simulink model "CAMFC2_04_Quad_03"  (R2018b)
settings: Solver=ode45  StartTime=0.0  StopTime=600  RelTol=1e-3  EnableMultiTasking=on
InitFcn:
  | constant_CAMFC2_04_Quad_03
values from neighbouring files (symbols this model uses):
  alpha = 0.1    [constant_CAMFC2_01_WMR01.m]    (also in constant_CAMFC2_04_Comp.m = 0.01; constant_CAMFC2_04_Quad_03.m; constant_CAMFC2_04_Simple.m = 0.01; constant_CAMFC2_04_Simple_DoubleIntegrator.m = 0.01)
  AN = [     0 1 0 0 ... (first row only)    [constant_CAMFC2_01_WMR01.m]    (also in constant_CAMFC2_04_Comp.m = [     0 1 0 0 1; constant_CAMFC2_04_Quad_03.m; constant_CAMFC2_04_Simple.m; constant_CAMFC2_04_Simple_DoubleIntegrator.m)
  B = eye(n)    [constant_CAMFC2_01_WMR01.m]    (also in constant_CAMFC2_04_Quad_03.m; constant_CAMFC2_Quad_New_02.m)
  BBT_inv = ((B'*B)^(-1))*B'    [constant_CAMFC2_04_Quad_03.m]    (also in constant_CAMFC2_Quad_New_02.m)
  Beta = 0.2    [constant_CAMFC2_04_Quad_03.m]    (also in constant_CAMFC2_Quad_New_02.m = 0.1)
  BN = [     1 0 0 0 ... (first row only)    [constant_CAMFC2_01_WMR01.m]    (also in constant_CAMFC2_04_Comp.m = [     0 0 0 0 0; constant_CAMFC2_04_Quad_03.m; constant_CAMFC2_04_Simple.m; constant_CAMFC2_04_Simple_DoubleIntegrator.m)
  Bv = eye(n0)    [constant_CAMFC2_04_Quad_03.m]
  BvBT_inv = ((Bv'*Bv)^(-1))*Bv'    [constant_CAMFC2_04_Quad_03.m]
  chi = [0 0 0 0 ... (first row only)    [constant_CAMFC2_01_WMR01.m]    (also in constant_CAMFC2_04_Comp.m = X_m*ones(n0,1); constant_CAMFC2_04_Quad_03.m = X_m*ones(n0,1); constant_CAMFC2_04_Simple.m = X_m*ones(n0,1); constant_CAMFC2_04_Simple_DoubleIntegrator.m = X_m*ones(n0,1))
  epsilon_struct = struct('data',epsilon_InitVal)    [constant_CAMFC2_01_WMR01.m]    (also in constant_CAMFC2_04_Comp.m; constant_CAMFC2_04_Quad_03.m; constant_CAMFC2_04_Simple.m; constant_CAMFC2_04_Simple_DoubleIntegrator.m)
  gama1 = 1e4*diag([1e-6*ones(2,1);1e0*ones(2,1)])    [constant_CAMFC2_01_WMR01.m]    (also in constant_CAMFC2_04_Comp.m = 1e+3*diag([1e-6;1e-0]); constant_CAMFC2_04_Quad_03.m = 1e+2*diag(1e-0*ones(n0,1)); constant_CAMFC2_04_Simple.m = 1e+2*diag([1e-0;1e-0]); constant_CAMFC2_04_Simple_Formation.m = 1e+2*diag([1e-0;1e-0]))
  gama2 = 1e-2*diag([1e-6*ones(2,1);1e0*ones(2,1)])    [constant_CAMFC2_01_WMR01.m]    (also in constant_CAMFC2_04_Comp.m = 1e+0*diag([1e-6;1e-0]); constant_CAMFC2_04_Quad_03.m = 1e+0*diag(1e-0*ones(n0,1)); constant_CAMFC2_04_Simple.m = 1e+1*diag([1e-0;1e-0]); constant_CAMFC2_04_Simple_Formation.m = 1e+1*diag([1e-0;1e-0]))
  gamma_0 = 1e+0*diag([1e-0*ones(n0,1);1e-0*ones(n0,1)])    [constant_CAMFC2_04_Quad_03.m]    (also in constant_CAMFC2_Quad_New_02.m = 1e-2*diag([1e-6*ones(n0,1);1e-0*ones(n0,1)]))
  gamma_0v = 1e-0*diag(1e-0*ones(n0,1))    [constant_CAMFC2_04_Quad_03.m]
  gamma_1 = 1e+2*diag([1e-0*ones(n0,1);1e-0*ones(n0,1)])    [constant_CAMFC2_04_Quad_03.m]    (also in constant_CAMFC2_Quad_New_02.m = 1e+1*diag([1e-6*ones(n0,1);1e-0*ones(n0,1)]))
  gamma_1v = 1e+2*diag(1e-0*ones(n0,1))    [constant_CAMFC2_04_Quad_03.m]
  ge = 9.81    [constant_CAMFC2_04_Comp.m]    (also in constant_CAMFC2_04_Quad_03.m; constant_CAMFC2_04_Simple.m; constant_CAMFC2_04_Simple_DoubleIntegrator.m; constant_CAMFC2_04_Simple_DoubleIntegrator_02.m)
  H = L + BN    [constant_CAMFC2_01_WMR01.m]    (also in constant_CAMFC2_04_Comp.m; constant_CAMFC2_04_Quad_03.m; constant_CAMFC2_04_Simple.m; constant_CAMFC2_04_Simple_DoubleIntegrator.m)
  J = 0.01    [constant_CAMFC2_01_WMR01.m]    (also in constant_CAMFC2_04_Quad_03.m = 1.0e-3 * diag([1 1 2],0); constant_CAMFC2_Quad_New_02.m = 1.2416e-3 * diag([1 1 2],0))
  k1 = 1    [constant_CAMFC2_01_WMR01.m]    (also in constant_CAMFC2_04_Comp.m; constant_CAMFC2_04_Quad_03.m = 50; constant_CAMFC2_04_Simple.m; constant_CAMFC2_04_Simple_DoubleIntegrator.m)
  k2 = 1    [constant_CAMFC2_01_WMR01.m]    (also in constant_CAMFC2_04_Comp.m; constant_CAMFC2_04_Quad_03.m; constant_CAMFC2_04_Simple.m; constant_CAMFC2_04_Simple_DoubleIntegrator.m)
  Ka = 0.1    [constant_CAMFC2_04_Quad_03.m]    (also in constant_CAMFC2_Quad_New_02.m = 0.01)
  Kd = 0.1    [constant_CAMFC2_04_Quad_03.m]    (also in constant_CAMFC2_Quad_New_02.m = 0.01)
  m = 6    [constant_CAMFC2_04_Quad_03.m]    (also in constant_CAMFC2_Quad_New_02.m)
  M = 1    [constant_CAMFC2_01_WMR01.m]    (also in constant_CAMFC2_04_Quad_03.m = 2; constant_CAMFC2_Quad_New_02.m = 2)
  N = 4    [constant_CAMFC2_01_WMR01.m]    (also in constant_CAMFC2_04_Comp.m = 5; constant_CAMFC2_04_Quad_03.m; constant_CAMFC2_04_Simple.m; constant_CAMFC2_04_Simple_DoubleIntegrator.m)
  n = 4    [constant_CAMFC2_01_WMR01.m]    (also in constant_CAMFC2_04_Comp.m = 2; constant_CAMFC2_04_Quad_03.m = 6; constant_CAMFC2_04_Simple.m = 2; constant_CAMFC2_04_Simple_DoubleIntegrator.m = 2)
  n0 = 2    [constant_CAMFC2_01_WMR01.m]    (also in constant_CAMFC2_04_Comp.m = 1; constant_CAMFC2_04_Quad_03.m = 3; constant_CAMFC2_04_Simple.m; constant_CAMFC2_04_Simple_DoubleIntegrator.m = 1)
  noise_amp = 0.1    [constant_CAMFC2_04_Quad_03.m]
  noise_frq = 1    [constant_CAMFC2_04_Quad_03.m]
  Observer_Gain = 100    [constant_CAMFC2_01_WMR01.m]    (also in constant_CAMFC2_04_Comp.m = 10; constant_CAMFC2_04_Quad_03.m = 1; constant_CAMFC2_04_Simple.m; constant_CAMFC2_04_Simple_DoubleIntegrator.m)
  Observer_Gain1 = 100    [constant_CAMFC2_01_WMR01.m]    (also in constant_CAMFC2_04_Comp.m = 10; constant_CAMFC2_04_Quad_03.m = 1; constant_CAMFC2_04_Simple.m; constant_CAMFC2_04_Simple_DoubleIntegrator.m)
  P_struct = struct('data',P_InitVal)    [constant_CAMFC2_01_WMR01.m]    (also in constant_CAMFC2_04_Comp.m; constant_CAMFC2_04_Quad_03.m; constant_CAMFC2_04_Simple.m; constant_CAMFC2_04_Simple_DoubleIntegrator.m)
  Q = 1e-0*eye(n)    [constant_CAMFC2_01_WMR01.m]    (also in constant_CAMFC2_04_Comp.m = 1.0e+2*eye(n); constant_CAMFC2_04_Quad_03.m = 1e-0*eye(n0); constant_CAMFC2_04_Simple.m = 1.0e+1*eye(n); constant_CAMFC2_04_Simple_Formation.m = 1.0e+1*eye(n))
  QR = 1e-0*eye(n)    [constant_CAMFC2_04_Quad_03.m]    (also in constant_CAMFC2_Quad_New_02.m = 1e+0*eye(n))
  Qv = 1e-0*eye(n0)    [constant_CAMFC2_04_Quad_03.m]
  R = 1e-0*eye(n)    [constant_CAMFC2_01_WMR01.m]    (also in constant_CAMFC2_04_Quad_03.m; constant_CAMFC2_Quad_New_02.m = 1e+0*eye(n))
  r_formX = 1.0    (= 1)    [constant_CAMFC2_04_Quad_03.m]    (also in constant_CAMFC2_Quad_New_02.m)
  r_formY = 1.0    (= 1)    [constant_CAMFC2_04_Quad_03.m]    (also in constant_CAMFC2_Quad_New_02.m)
  r_formZ = 0.5    [constant_CAMFC2_04_Quad_03.m]    (also in constant_CAMFC2_Quad_New_02.m = 1)
  rho1 = 1e-1    (= 0.1)    [constant_CAMFC2_01_WMR01.m]    (also in constant_CAMFC2_04_Comp.m = 1; constant_CAMFC2_04_Quad_03.m = 1; constant_CAMFC2_04_Simple.m = 1; constant_CAMFC2_04_Simple_DoubleIntegrator.m = 1)
  rho2 = 1e-3    (= 0.001)    [constant_CAMFC2_01_WMR01.m]    (also in constant_CAMFC2_04_Comp.m = 1; constant_CAMFC2_04_Quad_03.m = 1; constant_CAMFC2_04_Simple.m = 1; constant_CAMFC2_04_Simple_DoubleIntegrator.m = 10)
  rho_0 = 1e-0    (= 1)    [constant_CAMFC2_04_Quad_03.m]    (also in constant_CAMFC2_Quad_New_02.m = 0.01)
  rho_0v = 1e-0    (= 1)    [constant_CAMFC2_04_Quad_03.m]
  rho_1 = 1e-0    (= 1)    [constant_CAMFC2_04_Quad_03.m]    (also in constant_CAMFC2_Quad_New_02.m = 0.01)
  rho_1v = 1e-0    (= 1)    [constant_CAMFC2_04_Quad_03.m]
  Rv = 1e-0*eye(n0)    [constant_CAMFC2_04_Quad_03.m]
  T_struct = struct('data',T_InitVal)    [constant_CAMFC2_01_WMR01.m]    (also in constant_CAMFC2_04_Comp.m; constant_CAMFC2_04_Quad_03.m; constant_CAMFC2_04_Simple.m; constant_CAMFC2_04_Simple_DoubleIntegrator.m)
  Upsilon_M = Upsilon_m*ones(n,1)    [constant_CAMFC2_01_WMR01.m]    (also in constant_CAMFC2_04_Comp.m; constant_CAMFC2_04_Quad_03.m = Upsilon_m*ones(n0,1); constant_CAMFC2_04_Simple.m; constant_CAMFC2_04_Simple_DoubleIntegrator.m)
  Vel_limit = 100    [constant_CAMFC2_04_Quad_03.m]
(part 1 of 4)
settings Model: ExtModeTrigDuration=100  Creator=hp  LastModifiedBy=asafae
settings DataIOCC: LimitDataPoints=on  SaveFinalState=on  SaveFormat=StructureWithTime  SaveOutput=off  SaveState=on  StateSaveName=tmp_raccel_xout  SignalLoggingName=tmp_raccel_logsout
settings OptimizationCC: EfficientMapNaN2IntZero=off  LifeSpan=inf
settings DebuggingCC: UnderspecifiedInitializationDetection=Classic  MergeDetectMultiDrivingBlocksExec=none  SFUnexpectedBacktrackingDiag=warning  SFNoUnconditionalDefaultTransitionDiag=warning  SFExecutionAtInitializationDiag=none
settings HardwareCC: ProdBitPerPointer=32  ProdBitPerSizeT=32  ProdBitPerPtrDiffT=32  ProdLargestAtomicFloat=None  ProdIntDivRoundTo=Undefined  ProdEndianess=Unspecified  ProdWordSize=32  ProdHWDeviceType=32-bit Generic  TargetBitPerPointer=64  TargetBitPerSizeT=64  TargetBitPerPtrDiffT=64  TargetLongLongMode=on  TargetIntDivRoundTo=Zero  TargetEndianess=LittleEndian  TargetWordSize=64  TargetHWDeviceType=MATLAB Host  ProdEqTarget=off
settings ModelReferenceCC: PropagateSignalLabelsOutOfModel=off
settings SFSimCC: SimUseLocalCustomCode=off
settings RTWCC: SystemTargetFile=raccel.tlc  TemplateMakefile=raccel_default_tmf  RTWVerbose=off  RTWUseLocalCustomCode=off  RTWUseSimCustomCode=on
settings CodeAppCC: GenerateComments=off  MaxIdLength=128  MangleLength=10  SimulinkBlockComments=off
settings RaccelTargetCC: GeneratePreprocessorConditionals=Use local settings  MultiInstanceERTCode=off  PreserveStateflowLocalDataDimensions=off  ExtModeMexArgs='', 0, 54523  ENABLE_SLEXEC_SSBRIDGE=0  RTWCAPIParams=on
settings ConfigComp: CovMetricSettings=dw  CovHtmlReporting=on  CovSaveCumulativeToWorkspaceVar=on  CovSaveSingleToWorkspaceVar=on  CovExternalEMLEnable=off

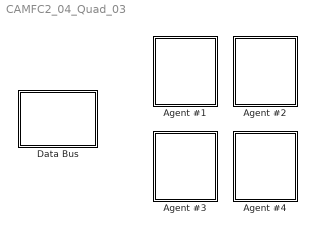
== system CAMFC2_04_Quad_03 ==
  Agent #1 : Subsystem
  Agent #2 : Subsystem
  Agent #3 : Subsystem
  Agent #4 : Subsystem
  "Data Bus " : Subsystem

== system CAMFC2_04_Quad_03/Agent #1 ==
  Agent # : Constant
  Decenteralized Cooperaive Controller #1 : Subsystem
  Plant #1 : Subsystem
  wires:
  Agent #/1 -> Decenteralized Cooperaive Controller #1/1(Agent No.)
  Decenteralized Cooperaive Controller #1/1(u1) -> Plant #1/1(U)

== system CAMFC2_04_Quad_03/Agent #2 ==
  Agent # : Constant  Value=2
  Decenteralized Cooperaive Controller #2 : Subsystem
  Plant #2 : Subsystem
  wires:
  Decenteralized Cooperaive Controller #2/1(u2) -> Plant #2/1(U)
  Agent #/1 -> Decenteralized Cooperaive Controller #2/1(Agent No.)

== system CAMFC2_04_Quad_03/Agent #3 ==
  Agent # : Constant  Value=3
  Decenteralized Cooperaive Controller #3 : Subsystem
  Plant #3 : Subsystem
  wires:
  Agent #/1 -> Decenteralized Cooperaive Controller #3/1(Agent No.)
  Decenteralized Cooperaive Controller #3/1(u3) -> Plant #3/1(U)

== system CAMFC2_04_Quad_03/Agent #4 ==
  Agent # : Constant  Value=4
  Decenteralized Cooperaive Controller #4 : Subsystem
  Plant #4 : Subsystem
  wires:
  Decenteralized Cooperaive Controller #4/1(u4) -> Plant #4/1(U)
  Agent #/1 -> Decenteralized Cooperaive Controller #4/1(Agent No.)

== system CAMFC2_04_Quad_03/Data Bus  ==
  Observers Log : Subsystem
  Reference Trajectory : Subsystem
  Rotational Log : Subsystem
  Scope26 : Scope
  Translational Log : Subsystem
  Velocity Log : Subsystem
  tag scope: x0=global
  wires:
  Reference Trajectory/1(X0) -> [x0], Scope26/1

== system CAMFC2_04_Quad_03/Agent #1/Decenteralized Cooperaive Controller #1 ==
  Agent No. : Inport
  Controller Interpreter #1 : MATLAB Function  TreatAsAtomicUnit=on
  Controller to Motors #1 : MATLAB Function  TreatAsAtomicUnit=on
  Cooperative Position Controller #1 : Subsystem
  Rotational AMFC #1 : Subsystem
  Scope : Scope
  Velocity AMFC #1 : Subsystem
  u1 : Outport
  tag scope: u1=global
  wires:
  Controller Interpreter #1/2(PHI_d_i) -> Scope/1, Rotational AMFC #1/1(x_rd)
  Controller Interpreter #1/1(uT_i) -> Controller to Motors #1/1(uT)
  Rotational AMFC #1/1(ur) -> Controller to Motors #1/2(uR)
  Controller to Motors #1/1(u) -> u1/1, [u1]
  [x1_R] -> Rotational AMFC #1/2(X)
  Agent No./1 -> Cooperative Position Controller #1/1(Agent #)
  Velocity AMFC #1/1(ut) -> Controller Interpreter #1/1(ut_i)
  Cooperative Position Controller #1/1(U1) -> Velocity AMFC #1/1(x_rd)
  [x1_TV] -> Velocity AMFC #1/2(X)

== system CAMFC2_04_Quad_03/Agent #1/Plant #1 ==
  U : Inport
  Clock : Clock
  Integrator : Integrator  InitialCondition=zeros(n0,1)
  Integrator1 : Integrator  InitialCondition=zeros(n,1)
  Integrator2 : Integrator  InitialCondition=zeros(n0,1)
  MATLAB Function : MATLAB Function  TreatAsAtomicUnit=on
  tag scope: x1_R=global, x1_TP=global, x1_TV=global
  wires:
  Clock/1 -> MATLAB Function/4(t)
  MATLAB Function/1(DP) -> Integrator/1
  Integrator/1 -> [x1_TP]
  U/1 -> MATLAB Function/3(U)
  Integrator1/1 -> [x1_R], MATLAB Function/2(XR)
  MATLAB Function/3(DXR) -> Integrator1/1
  MATLAB Function/2(Dv) -> Integrator2/1
  Integrator2/1 -> MATLAB Function/1(XT_V), [x1_TV]

== system CAMFC2_04_Quad_03/Agent #2/Decenteralized Cooperaive Controller #2 ==
  Agent No. : Inport
  Controller Interpreter #2 : MATLAB Function  TreatAsAtomicUnit=on
  Controller to Motors #2 : MATLAB Function  TreatAsAtomicUnit=on
  Cooperative Position Controller #2 : Subsystem
  Rotational AMFC #2 : Subsystem
  Scope : Scope
  Velocity AMFC #2 : Subsystem
  u2 : Outport
  tag scope: u2=global
  wires:
  [x2_TV] -> Velocity AMFC #2/2(X)
  Cooperative Position Controller #2/1(U2) -> Velocity AMFC #2/1(x_rd)
  Velocity AMFC #2/1(ut) -> Controller Interpreter #2/1(ut_i)
  Agent No./1 -> Cooperative Position Controller #2/1(Agent #)
  [x2_R] -> Rotational AMFC #2/2(X)
  Controller to Motors #2/1(u) -> [u2], u2/1
  Rotational AMFC #2/1(ur) -> Controller to Motors #2/2(uR)
  Controller Interpreter #2/1(uT_i) -> Controller to Motors #2/1(uT)
  Controller Interpreter #2/2(PHI_d_i) -> Scope/1, Rotational AMFC #2/1(x_rd)

== system CAMFC2_04_Quad_03/Agent #2/Plant #2 ==
  U : Inport
  Clock : Clock
  Integrator : Integrator  InitialCondition=zeros(n0,1)
  Integrator1 : Integrator  InitialCondition=zeros(n,1)
  Integrator2 : Integrator  InitialCondition=zeros(n0,1)
  MATLAB Function : MATLAB Function  TreatAsAtomicUnit=on
  tag scope: x2_R=global, x2_TP=global, x2_TV=global
  wires:
  Integrator2/1 -> MATLAB Function/1(XT_V), [x2_TV]
  MATLAB Function/2(Dv) -> Integrator2/1
  MATLAB Function/3(DXR) -> Integrator1/1
  Integrator1/1 -> MATLAB Function/2(XR), [x2_R]
  U/1 -> MATLAB Function/3(U)
  Integrator/1 -> [x2_TP]
  MATLAB Function/1(DP) -> Integrator/1
  Clock/1 -> MATLAB Function/4(t)

== system CAMFC2_04_Quad_03/Agent #3/Decenteralized Cooperaive Controller #3 ==
  Agent No. : Inport
  Controller Interpreter #3 : MATLAB Function  TreatAsAtomicUnit=on
  Controller to Motors #3 : MATLAB Function  TreatAsAtomicUnit=on
  Cooperative Position Controller #3 : Subsystem
  Rotational AMFC #3 : Subsystem
  Scope : Scope
  Velocity AMFC #3 : Subsystem
  u3 : Outport
  tag scope: u3=global
  wires:
  Controller Interpreter #3/2(PHI_d_i) -> Scope/1, Rotational AMFC #3/1(x_rd)
  Controller Interpreter #3/1(uT_i) -> Controller to Motors #3/1(uT)
  Rotational AMFC #3/1(ur) -> Controller to Motors #3/2(uR)
  Controller to Motors #3/1(u) -> u3/1, [u3]
  [x3_R] -> Rotational AMFC #3/2(X)
  Agent No./1 -> Cooperative Position Controller #3/1(Agent #)
  Velocity AMFC #3/1(ur) -> Controller Interpreter #3/1(ut_i)
  Cooperative Position Controller #3/1(U3) -> Velocity AMFC #3/1(x_rd)
  [x3_TV] -> Velocity AMFC #3/2(X)

== system CAMFC2_04_Quad_03/Agent #3/Plant #3 ==
  U : Inport
  Clock : Clock
  Integrator : Integrator  InitialCondition=zeros(n0,1)
  Integrator1 : Integrator  InitialCondition=zeros(n,1)
  Integrator2 : Integrator  InitialCondition=zeros(n0,1)
  MATLAB Function : MATLAB Function  TreatAsAtomicUnit=on
  tag scope: x3_R=global, x3_TP=global, x3_TV=global
  wires:
  Clock/1 -> MATLAB Function/4(t)
  MATLAB Function/1(DP) -> Integrator/1
  Integrator/1 -> [x3_TP]
  U/1 -> MATLAB Function/3(U)
  Integrator1/1 -> MATLAB Function/2(XR), [x3_R]
  MATLAB Function/3(DXR) -> Integrator1/1
  MATLAB Function/2(Dv) -> Integrator2/1
  Integrator2/1 -> MATLAB Function/1(XT_V), [x3_TV]

== system CAMFC2_04_Quad_03/Agent #4/Decenteralized Cooperaive Controller #4 ==
  Agent No. : Inport
  Controller Interpreter #4 : MATLAB Function  TreatAsAtomicUnit=on
  Controller to Motors #4 : MATLAB Function  TreatAsAtomicUnit=on
  Cooperative Position Controller #4 : Subsystem
  Rotational AMFC #4 : Subsystem
  Scope : Scope
  Velocity AMFC #4 : Subsystem
  u4 : Outport
  tag scope: u4=global
  wires:
  [x4_TV] -> Velocity AMFC #4/2(X)
  Cooperative Position Controller #4/1(U4) -> Velocity AMFC #4/1(x_rd)
  Velocity AMFC #4/1(ur) -> Controller Interpreter #4/1(ut_i)
  Agent No./1 -> Cooperative Position Controller #4/1(Agent #)
  [x4_R] -> Rotational AMFC #4/2(X)
  Controller to Motors #4/1(u) -> [u4], u4/1
  Rotational AMFC #4/1(ur) -> Controller to Motors #4/2(uR)
  Controller Interpreter #4/1(uT_i) -> Controller to Motors #4/1(uT)
  Controller Interpreter #4/2(PHI_d_i) -> Scope/1, Rotational AMFC #4/1(x_rd)

== system CAMFC2_04_Quad_03/Agent #4/Plant #4 ==
  U : Inport
  Clock : Clock
  Integrator : Integrator  InitialCondition=zeros(n0,1)
  Integrator1 : Integrator  InitialCondition=zeros(n,1)
  Integrator2 : Integrator  InitialCondition=zeros(n0,1)
  MATLAB Function : MATLAB Function  TreatAsAtomicUnit=on
  tag scope: x4_R=global, x4_TP=global, x4_TV=global
  wires:
  Integrator2/1 -> MATLAB Function/1(XT_V), [x4_TV]
  MATLAB Function/2(Dv) -> Integrator2/1
  MATLAB Function/3(DXR) -> Integrator1/1
  Integrator1/1 -> MATLAB Function/2(XR), [x4_R]
  U/1 -> MATLAB Function/3(U)
  Integrator/1 -> [x4_TP]
  MATLAB Function/1(DP) -> Integrator/1
  Clock/1 -> MATLAB Function/4(t)

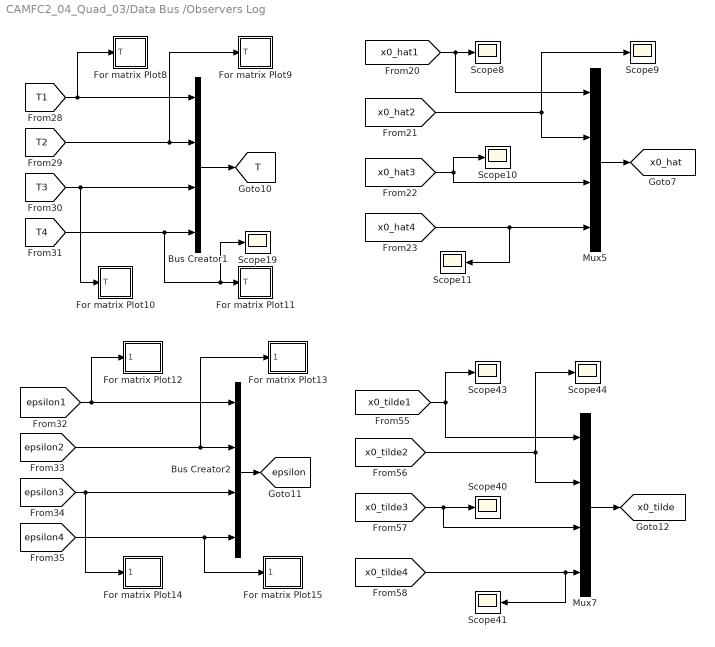
== system CAMFC2_04_Quad_03/Data Bus /Observers Log ==
  Bus Creator1 : BusCreator  Inputs=4  OutDataTypeStr=Bus: T_bus
  Bus Creator2 : BusCreator  Inputs=4  OutDataTypeStr=Bus: epsilon_bus
  For matrix Plot10 : Subsystem
  For matrix Plot11 : Subsystem
  For matrix Plot12 : Subsystem
  For matrix Plot13 : Subsystem
  For matrix Plot14 : Subsystem
  For matrix Plot15 : Subsystem
  For matrix Plot8 : Subsystem
  For matrix Plot9 : Subsystem
  Mux5 : Mux
  Mux7 : Mux
  Scope{8..11,19,40..41,43..44} (9 alike) : Scope
  tag scope: T=global, epsilon=global, x0_hat=global, x0_tilde=global
  wires:
  [epsilon4] -> For matrix Plot15/1(epsilon), Bus Creator2/4
  [x0_tilde1] -> Scope43/1, Mux7/1
  [epsilon1] -> For matrix Plot12/1(epsilon), Bus Creator2/1
  [T2] -> For matrix Plot9/1(T), Bus Creator1/2
  Mux7/1 -> [x0_tilde]
  [x0_tilde3] -> Mux7/3, Scope40/1
  Bus Creator2/1 -> [epsilon]
  [T3] -> For matrix Plot10/1(T), Bus Creator1/3
  [x0_tilde2] -> Scope44/1, Mux7/2
  [epsilon3] -> For matrix Plot14/1(epsilon), Bus Creator2/3
  [T4] -> Scope19/1, For matrix Plot11/1(T), Bus Creator1/4
  [x0_tilde4] -> Scope41/1, Mux7/4
  [epsilon2] -> For matrix Plot13/1(epsilon), Bus Creator2/2
  [T1] -> For matrix Plot8/1(T), Bus Creator1/1
  Bus Creator1/1 -> [T]
  [x0_hat1] -> Scope8/1, Mux5/1
  [x0_hat4] -> Mux5/4, Scope11/1
  [x0_hat3] -> Scope10/1, Mux5/3
  [x0_hat2] -> Scope9/1, Mux5/2
  Mux5/1 -> [x0_hat]

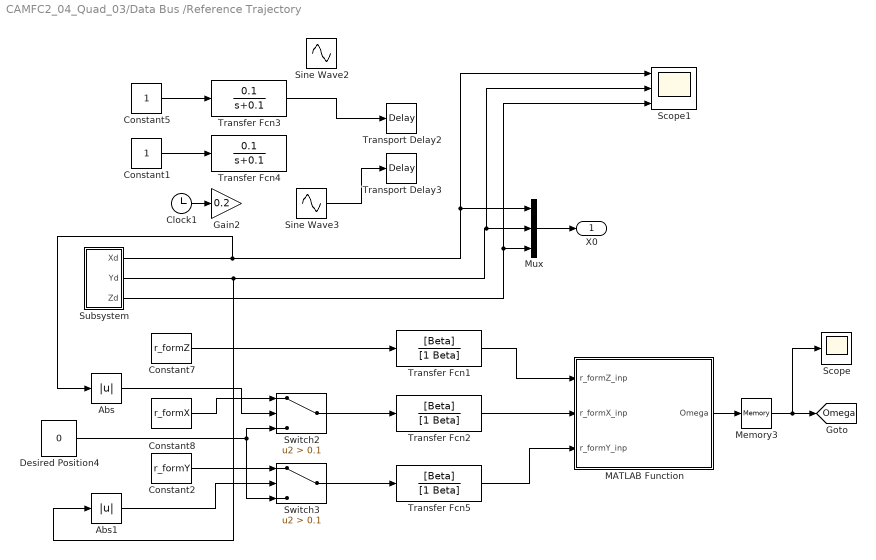
== system CAMFC2_04_Quad_03/Data Bus /Reference Trajectory ==
  Abs : Abs
  Abs1 : Abs
  Clock1 : Clock
  Constant1 : Constant
  Constant2 : Constant  Value=r_formY
  Constant5 : Constant
  Constant7 : Constant  Value=r_formZ
  Constant8 : Constant  Value=r_formX
  Desired Position4 : Constant  Value=0  VectorParams1D=off
  Gain2 : Gain  Gain=0.2
  MATLAB Function : MATLAB Function  TreatAsAtomicUnit=on
  Memory3 : Memory  InitialCondition=zeros(N+1,n0)
  Mux : Mux  Inputs=3
  Scope : Scope
  Scope1 : Scope  NumInputPorts=3
  Sine Wave2 : Sin  Amplitude=3  Bias=-3  Frequency=0.1  Phase=pi/2  SampleTime=0
  Sine Wave3 : Sin  Amplitude=3  Frequency=0.1  SampleTime=0
  Subsystem : Subsystem
  Switch2 : Switch  Criteria=u2 > Threshold  Threshold=0.1
  Switch3 : Switch  Criteria=u2 > Threshold  Threshold=0.1
  Transfer Fcn1 : TransferFcn  Numerator=[Beta]  Denominator=[1 Beta]
  Transfer Fcn2 : TransferFcn  Numerator=[Beta]  Denominator=[1 Beta]
  Transfer Fcn3 : TransferFcn  Numerator=[0.1]  Denominator=[1 0.1]
  Transfer Fcn4 : TransferFcn  Numerator=[0.1]  Denominator=[1 0.1]
  Transfer Fcn5 : TransferFcn  Numerator=[Beta]  Denominator=[1 Beta]
  Transport Delay2 : TransportDelay  DelayTime=20
  Transport Delay3 : TransportDelay  DelayTime=20
  X0 : Outport
  tag scope: Omega=global
  wires:
  Subsystem/1(Xd) -> Abs/1, Scope1/1, Mux/1
  Mux/1 -> X0/1
  MATLAB Function/1(Omega) -> Memory3/1
  Transfer Fcn1/1 -> MATLAB Function/1(r_formZ_inp)
  Transfer Fcn2/1 -> MATLAB Function/2(r_formX_inp)
  Constant5/1 -> Transfer Fcn3/1
  Clock1/1 -> Gain2/1
  Subsystem/2(Yd) -> Abs1/1, Scope1/2, Mux/2
  Constant1/1 -> Transfer Fcn4/1
  Sine Wave3/1 -> Transport Delay3/1
  Switch3/1 -> Transfer Fcn5/1
  Transfer Fcn5/1 -> MATLAB Function/3(r_formY_inp)
  Transfer Fcn3/1 -> Transport Delay2/1
  Switch2/1 -> Transfer Fcn2/1
  Constant7/1 -> Transfer Fcn1/1
  Subsystem/3(Zd) -> Scope1/3, Mux/3
  Abs/1 -> Switch2/2
  Constant8/1 -> Switch2/1
  Desired Position4/1 -> Switch2/3, Switch3/3
  Constant2/1 -> Switch3/1
  Abs1/1 -> Switch3/2
  Memory3/1 -> Scope/1, [Omega]

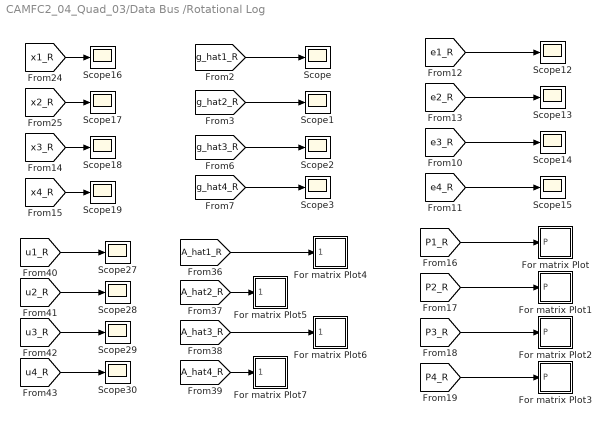
== system CAMFC2_04_Quad_03/Data Bus /Rotational Log ==
  For matrix Plot : Subsystem
  For matrix Plot1 : Subsystem
  For matrix Plot2 : Subsystem
  For matrix Plot3 : Subsystem
  For matrix Plot4 : Subsystem
  For matrix Plot5 : Subsystem
  For matrix Plot6 : Subsystem
  For matrix Plot7 : Subsystem
  Scope{,1..3,12..19,27..30} (16 alike) : Scope
  wires:
  [g_hat1_R] -> Scope/1
  [g_hat3_R] -> Scope2/1
  [g_hat2_R] -> Scope1/1
  [g_hat4_R] -> Scope3/1
  [e2_R] -> Scope13/1
  [P1_R] -> For matrix Plot/1(P)
  [e4_R] -> Scope15/1
  [P4_R] -> For matrix Plot3/1(P)
  [e3_R] -> Scope14/1
  [P3_R] -> For matrix Plot2/1(P)
  [e1_R] -> Scope12/1
  [P2_R] -> For matrix Plot1/1(P)
  [A_hat4_R] -> For matrix Plot7/1(A_hat)
  [A_hat2_R] -> For matrix Plot5/1(A_hat)
  [A_hat1_R] -> For matrix Plot4/1(A_hat)
  [A_hat3_R] -> For matrix Plot6/1(A_hat)
  [x4_R] -> Scope19/1
  [x2_R] -> Scope17/1
  [x3_R] -> Scope18/1
  [x1_R] -> Scope16/1
  [u2_R] -> Scope28/1
  [u1_R] -> Scope27/1
  [u4_R] -> Scope30/1
  [u3_R] -> Scope29/1

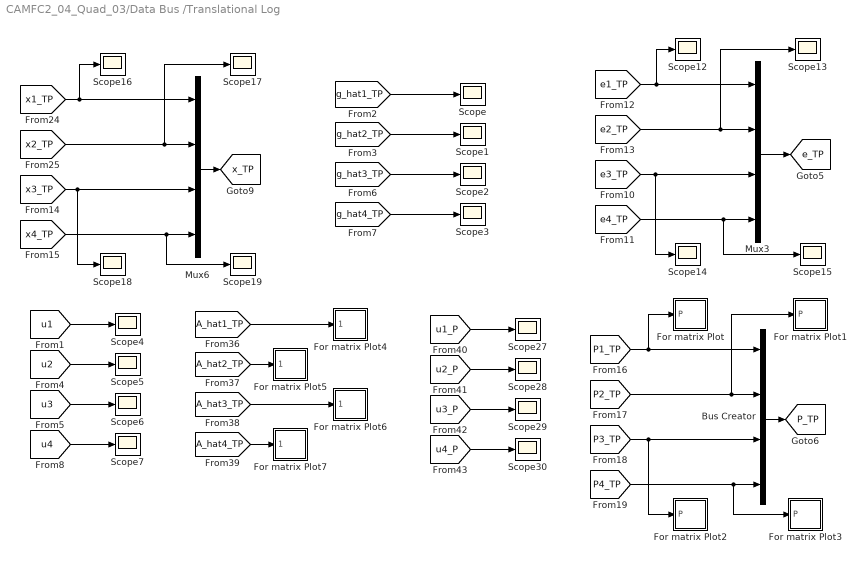
== system CAMFC2_04_Quad_03/Data Bus /Translational Log ==
  Bus Creator : BusCreator  Inputs=4  OutDataTypeStr=Bus: P_bus
  For matrix Plot : Subsystem
  For matrix Plot1 : Subsystem
  For matrix Plot2 : Subsystem
  For matrix Plot3 : Subsystem
  For matrix Plot4 : Subsystem
  For matrix Plot5 : Subsystem
  For matrix Plot6 : Subsystem
  For matrix Plot7 : Subsystem
  Mux3 : Mux
  Mux6 : Mux
  Scope{,1..7,12..19,27..30} (20 alike) : Scope
  tag scope: P_TP=global, e_TP=global, x_TP=global
  wires:
  [A_hat3_TP] -> For matrix Plot6/1(A_hat)
  [A_hat1_TP] -> For matrix Plot4/1(A_hat)
  [A_hat2_TP] -> For matrix Plot5/1(A_hat)
  [A_hat4_TP] -> For matrix Plot7/1(A_hat)
  [P2_TP] -> For matrix Plot1/1(P), Bus Creator/2
  [e1_TP] -> Scope12/1, Mux3/1
  [P3_TP] -> For matrix Plot2/1(P), Bus Creator/3
  [e3_TP] -> Scope14/1, Mux3/3
  Bus Creator/1 -> [P_TP]
  [P4_TP] -> For matrix Plot3/1(P), Bus Creator/4
  [e4_TP] -> Mux3/4, Scope15/1
  [P1_TP] -> For matrix Plot/1(P), Bus Creator/1
  [e2_TP] -> Scope13/1, Mux3/2
  Mux3/1 -> [e_TP]
  [u2_P] -> Scope28/1
  [u3_P] -> Scope29/1
  [u1_P] -> Scope27/1
  [u4_P] -> Scope30/1
  [g_hat4_TP] -> Scope3/1
  [g_hat2_TP] -> Scope1/1
  [g_hat3_TP] -> Scope2/1
  [g_hat1_TP] -> Scope/1
  [x3_TP] -> Scope18/1, Mux6/3
  [x1_TP] -> Scope16/1, Mux6/1
  Mux6/1 -> [x_TP]
  [x4_TP] -> Mux6/4, Scope19/1
  [x2_TP] -> Scope17/1, Mux6/2
  [u4] -> Scope7/1
  [u1] -> Scope4/1
  [u3] -> Scope6/1
  [u2] -> Scope5/1

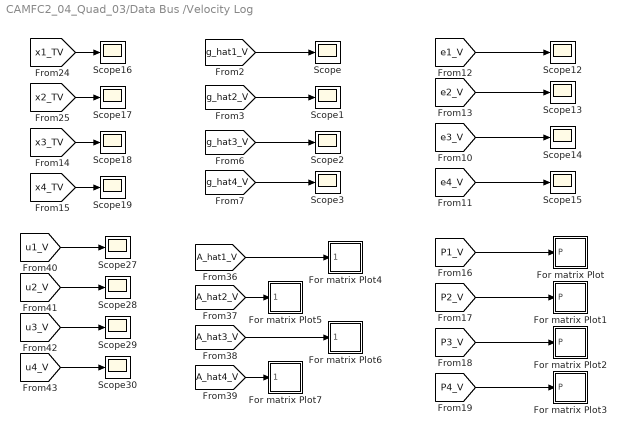
== system CAMFC2_04_Quad_03/Data Bus /Velocity Log ==
  For matrix Plot : Subsystem
  For matrix Plot1 : Subsystem
  For matrix Plot2 : Subsystem
  For matrix Plot3 : Subsystem
  For matrix Plot4 : Subsystem
  For matrix Plot5 : Subsystem
  For matrix Plot6 : Subsystem
  For matrix Plot7 : Subsystem
  Scope{,1..3,12..19,27..30} (16 alike) : Scope
  wires:
  [x1_TV] -> Scope16/1
  [x3_TV] -> Scope18/1
  [x2_TV] -> Scope17/1
  [x4_TV] -> Scope19/1
  [A_hat3_V] -> For matrix Plot6/1(A_hat)
  [A_hat1_V] -> For matrix Plot4/1(A_hat)
  [A_hat2_V] -> For matrix Plot5/1(A_hat)
  [A_hat4_V] -> For matrix Plot7/1(A_hat)
  [P2_V] -> For matrix Plot1/1(P)
  [e1_V] -> Scope12/1
  [P3_V] -> For matrix Plot2/1(P)
  [e3_V] -> Scope14/1
  [P4_V] -> For matrix Plot3/1(P)
  [e4_V] -> Scope15/1
  [P1_V] -> For matrix Plot/1(P)
  [e2_V] -> Scope13/1
  [g_hat4_V] -> Scope3/1
  [g_hat2_V] -> Scope1/1
  [g_hat3_V] -> Scope2/1
  [g_hat1_V] -> Scope/1
  [u2_V] -> Scope28/1
  [u1_V] -> Scope27/1
  [u4_V] -> Scope30/1
  [u3_V] -> Scope29/1

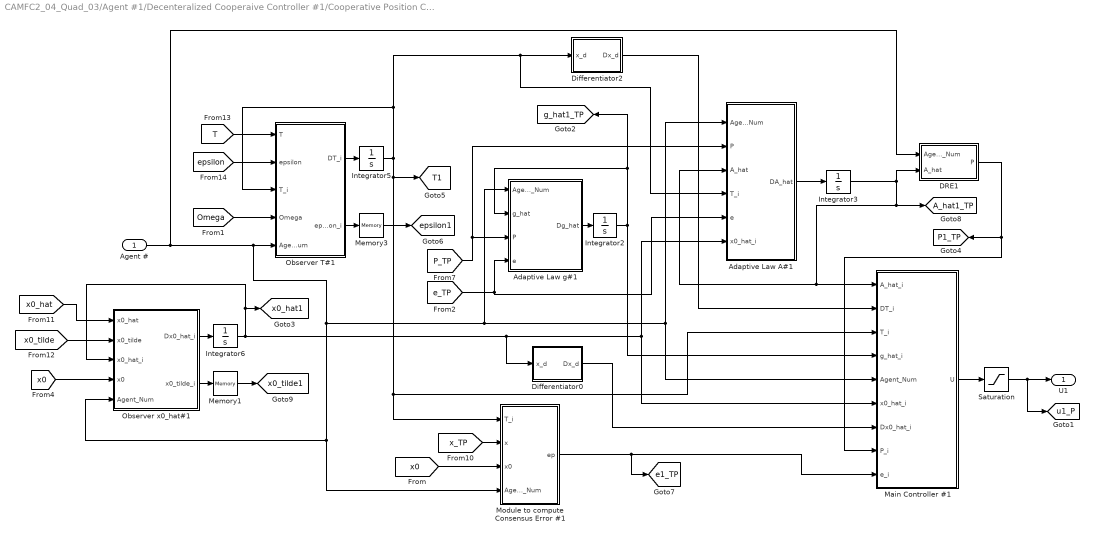
== system CAMFC2_04_Quad_03/Agent #1/Decenteralized Cooperaive Controller #1/Cooperative Position Controller #1 ==
  Agent # : Inport
  Adaptive Law A#1 : MATLAB Function  TreatAsAtomicUnit=on
  Adaptive Law g#1 : MATLAB Function  TreatAsAtomicUnit=on
  DRE1 : Subsystem
  Differentiator0 : Subsystem
  Differentiator2 : Subsystem
  Integrator2 : Integrator  InitialCondition=zeros(n0,1)
  Integrator3 : Integrator  InitialCondition=zeros(n0)
  Integrator5 : Integrator  InitialCondition=zeros(N+1,n0)
  Integrator6 : Integrator  InitialCondition=zeros(n0,1)
  Main Controller #1 : MATLAB Function  TreatAsAtomicUnit=on
  Memory1 : Memory  InitialCondition=zeros(n0,1)
  Memory3 : Memory  InitialCondition=zeros(N+1,n0)
  Module to compute Consensus Error #1 : MATLAB Function  TreatAsAtomicUnit=on
  Observer T#1 : MATLAB Function  TreatAsAtomicUnit=on
  Observer x0_hat#1 : MATLAB Function  TreatAsAtomicUnit=on
  Saturation : Saturate  UpperLimit=Vel_limit*ones(n0,1)  LowerLimit=-Vel_limit*ones(n0,1)
  U1 : Outport
  tag scope: A_hat1_TP=global, P1_TP=global, T1=global, e1_TP=global, epsilon1=global, g_hat1_TP=global, u1_P=global, x0_hat1=global, x0_tilde1=global
  wires:
  [x_TP] -> Module to compute Consensus Error #1/2(x)
  [x0] -> Module to compute Consensus Error #1/3(x0)
  Differentiator2/1(Dx_d) -> Main Controller #1/2(DT_i)
  [epsilon] -> Observer T#1/2(epsilon)
  [T] -> Observer T#1/1(T)
  Memory3/1 -> [epsilon1]
  Observer T#1/2(epsilon_i) -> Memory3/1
  Integrator5/1 -> [T1], Module to compute Consensus Error #1/1(T_i), Main Controller #1/3(T_i), Adaptive Law A#1/4(T_i), Differentiator2/1(x_d), Observer T#1/3(T_i)
  Observer T#1/1(DT_i) -> Integrator5/1
  Module to compute Consensus Error #1/1(ep) -> [e1_TP], Main Controller #1/9(e_i)
  Integrator3/1 -> DRE1/2(A_hat), Main Controller #1/1(A_hat_i), Adaptive Law A#1/3(A_hat), [A_hat1_TP]
  [e_TP] -> Adaptive Law A#1/5(e), Adaptive Law g#1/4(e)
  [P_TP] -> Adaptive Law A#1/2(P), Adaptive Law g#1/3(P)
  DRE1/1(P) -> Main Controller #1/8(P_i), [P1_TP]
  Integrator2/1 -> Main Controller #1/4(g_hat_i), Adaptive Law g#1/2(g_hat), [g_hat1_TP]
  Adaptive Law g#1/1(Dg_hat) -> Integrator2/1
  Adaptive Law A#1/1(DA_hat) -> Integrator3/1
  Agent #/1 -> DRE1/1(Agent_Num), Observer T#1/5(Agent_Num), Observer x0_hat#1/5(Agent_Num), Module to compute Consensus Error #1/4(Agent_Num), Adaptive Law g#1/1(Agent_Num), Adaptive Law A#1/1(Agent_Num), Main Controller #1/5(Agent_Num)
  Observer x0_hat#1/2(x0_tilde_i) -> Memory1/1
  Memory1/1 -> [x0_tilde1]
  Observer x0_hat#1/1(Dx0_hat_i) -> Integrator6/1
  [x0_tilde] -> Observer x0_hat#1/2(x0_tilde)
  [x0] -> Observer x0_hat#1/4(x0)
  [x0_hat] -> Observer x0_hat#1/1(x0_hat)
  Integrator6/1 -> Observer x0_hat#1/3(x0_hat_i), [x0_hat1], Differentiator0/1(x_d), Main Controller #1/6(x0_hat_i), Adaptive Law A#1/6(x0_hat_i)
  Differentiator0/1(Dx_d) -> Main Controller #1/7(Dx0_hat_i)
  [Omega] -> Observer T#1/4(Omega)
  Main Controller #1/1(U) -> Saturation/1
  Saturation/1 -> [u1_P], U1/1

== system CAMFC2_04_Quad_03/Agent #1/Decenteralized Cooperaive Controller #1/Rotational AMFC #1 ==
  x_rd : Inport
  X : Inport  Port=2
  CARE : MATLAB Function  TreatAsAtomicUnit=on
  Differentiator : Subsystem
  Integrator : Integrator  InitialCondition=zeros(n)
  Integrator1 : Integrator  InitialCondition=eye(n)
  Integrator2 : Integrator  InitialCondition=zeros(n,1)
  Integrator3 : Integrator  InitialCondition=zeros(n,1)
  Memory : Memory  InitialCondition=zeros(m,1)
  Sum : Sum  Inputs=|++
  g-Estimator : MATLAB Function  TreatAsAtomicUnit=on
  g-Estimator1 : MATLAB Function  TreatAsAtomicUnit=on
  main : MATLAB Function  TreatAsAtomicUnit=on
  variable change : MATLAB Function  TreatAsAtomicUnit=on
  ur : Outport
  tag scope: A_hat1_R=global, P1_R=global, e1_R=global, g_hat1_R=global, u1_R=global
  wires:
  x_rd/1 -> variable change/2(Xd)
  X/1 -> variable change/1(X)
  CARE/1(DP) -> Integrator1/1
  Sum/1 -> main/1(sigma), g-Estimator/1(sigma), g-Estimator1/1(sigma)
  g-Estimator1/1(Da_hat) -> Integrator/1
  variable change/1(x_mod) -> main/7(x), g-Estimator1/2(x)
  Integrator1/1 -> g-Estimator1/3(P), CARE/1(P), [P1_R], g-Estimator/3(P), main/4(P)
  Integrator/1 -> [A_hat1_R], g-Estimator1/4(a_hat), CARE/2(a_hat), main/5(a_hat)
  g-Estimator/1(Dg_hat) -> Integrator2/1
  Differentiator/1(Dx_d) -> main/3(Dy_d)
  main/1(u) -> Memory/1, [u1_R], ur/1
  Integrator3/1 -> main/2(zeta), Sum/1
  variable change/2(xd_mod) -> Differentiator/1(x_d)
  variable change/3(e_mod) -> [e1_R], Integrator3/1, Sum/2
  Memory/1 -> variable change/3(u)
  Integrator2/1 -> main/6(g_hat), [g_hat1_R], g-Estimator/2(g_hat)

== system CAMFC2_04_Quad_03/Agent #1/Decenteralized Cooperaive Controller #1/Velocity AMFC #1 ==
  x_rd : Inport
  X : Inport  Port=2
  "A-Estimator " : MATLAB Function  TreatAsAtomicUnit=on
  CARE : MATLAB Function  TreatAsAtomicUnit=on
  Differentiator : Subsystem
  Integrator : Integrator  InitialCondition=zeros(n0)
  Integrator1 : Integrator  InitialCondition=eye(n0)
  Integrator2 : Integrator  InitialCondition=zeros(n0,1)
  Integrator3 : Integrator  InitialCondition=zeros(n0,1)
  Sum : Sum  Inputs=|++
  g-Estimator : MATLAB Function  TreatAsAtomicUnit=on
  main : MATLAB Function  TreatAsAtomicUnit=on
  variable change : MATLAB Function  TreatAsAtomicUnit=on
  ut : Outport
  tag scope: A_hat1_V=global, P1_V=global, e1_V=global, g_hat1_V=global, u1_V=global
  wires:
  Integrator2/1 -> main/6(g_hat), [g_hat1_V], g-Estimator/2(g_hat)
  variable change/3(e_mod) -> Integrator3/1, Sum/2, [e1_V]
  variable change/2(xd_mod) -> Differentiator/1(x_d)
  Integrator3/1 -> Sum/1, main/2(zeta)
  main/1(u) -> [u1_V], ut/1
  Differentiator/1(Dx_d) -> main/3(Dy_d)
  g-Estimator/1(Dg_hat) -> Integrator2/1
  Integrator/1 -> main/5(a_hat), CARE/2(a_hat), "A-Estimator "/4(a_hat), [A_hat1_V]
  Integrator1/1 -> main/4(P), g-Estimator/3(P), [P1_V], CARE/1(P), "A-Estimator "/3(P)
  variable change/1(x_mod) -> "A-Estimator "/2(x), main/7(x)
  "A-Estimator "/1(Da_hat) -> Integrator/1
  Sum/1 -> "A-Estimator "/1(sigma), g-Estimator/1(sigma), main/1(sigma)
  CARE/1(DP) -> Integrator1/1
  X/1 -> variable change/1(X)
  x_rd/1 -> variable change/2(Xd)

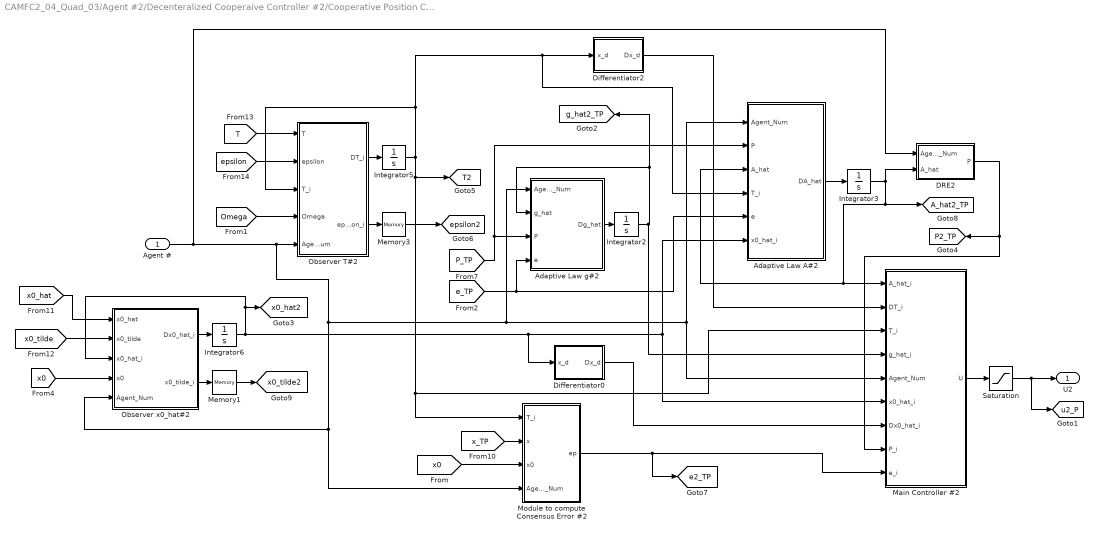
== system CAMFC2_04_Quad_03/Agent #2/Decenteralized Cooperaive Controller #2/Cooperative Position Controller #2 ==
  Agent # : Inport
  Adaptive Law A#2 : MATLAB Function  TreatAsAtomicUnit=on
  Adaptive Law g#2 : MATLAB Function  TreatAsAtomicUnit=on
  DRE2 : Subsystem
  Differentiator0 : Subsystem
  Differentiator2 : Subsystem
  Integrator2 : Integrator  InitialCondition=zeros(n0,1)
  Integrator3 : Integrator  InitialCondition=zeros(n0)
  Integrator5 : Integrator  InitialCondition=zeros(N+1,n0)
  Integrator6 : Integrator  InitialCondition=zeros(n0,1)
  Main Controller #2 : MATLAB Function  TreatAsAtomicUnit=on
  Memory1 : Memory  InitialCondition=zeros(n0,1)
  Memory3 : Memory  InitialCondition=zeros(N+1,n0)
  Module to compute Consensus Error #2 : MATLAB Function  TreatAsAtomicUnit=on
  Observer T#2 : MATLAB Function  TreatAsAtomicUnit=on
  Observer x0_hat#2 : MATLAB Function  TreatAsAtomicUnit=on
  Saturation : Saturate  UpperLimit=Vel_limit*ones(n0,1)  LowerLimit=-Vel_limit*ones(n0,1)
  U2 : Outport
  tag scope: A_hat2_TP=global, P2_TP=global, T2=global, e2_TP=global, epsilon2=global, g_hat2_TP=global, u2_P=global, x0_hat2=global, x0_tilde2=global
  wires:
  Main Controller #2/1(U) -> Saturation/1
  [Omega] -> Observer T#2/4(Omega)
  Differentiator0/1(Dx_d) -> Main Controller #2/7(Dx0_hat_i)
  Integrator6/1 -> Differentiator0/1(x_d), Adaptive Law A#2/6(x0_hat_i), Main Controller #2/6(x0_hat_i), [x0_hat2], Observer x0_hat#2/3(x0_hat_i)
  [x0_hat] -> Observer x0_hat#2/1(x0_hat)
  [x0] -> Observer x0_hat#2/4(x0)
  [x0_tilde] -> Observer x0_hat#2/2(x0_tilde)
  Observer x0_hat#2/1(Dx0_hat_i) -> Integrator6/1
  Memory1/1 -> [x0_tilde2]
  Observer x0_hat#2/2(x0_tilde_i) -> Memory1/1
  Agent #/1 -> Main Controller #2/5(Agent_Num), Adaptive Law A#2/1(Agent_Num), Adaptive Law g#2/1(Agent_Num), Module to compute Consensus Error #2/4(Agent_Num), Observer x0_hat#2/5(Agent_Num), Observer T#2/5(Agent_Num), DRE2/1(Agent_Num)
  Adaptive Law A#2/1(DA_hat) -> Integrator3/1
  Adaptive Law g#2/1(Dg_hat) -> Integrator2/1
  Integrator2/1 -> [g_hat2_TP], Adaptive Law g#2/2(g_hat), Main Controller #2/4(g_hat_i)
  DRE2/1(P) -> [P2_TP], Main Controller #2/8(P_i)
  [P_TP] -> Adaptive Law g#2/3(P), Adaptive Law A#2/2(P)
  [e_TP] -> Adaptive Law A#2/5(e), Adaptive Law g#2/4(e)
  Integrator3/1 -> Main Controller #2/1(A_hat_i), Adaptive Law A#2/3(A_hat), [A_hat2_TP], DRE2/2(A_hat)
  Module to compute Consensus Error #2/1(ep) -> [e2_TP], Main Controller #2/9(e_i)
  Observer T#2/1(DT_i) -> Integrator5/1
  Integrator5/1 -> Observer T#2/3(T_i), Differentiator2/1(x_d), Adaptive Law A#2/4(T_i), Main Controller #2/3(T_i), Module to compute Consensus Error #2/1(T_i), [T2]
  Observer T#2/2(epsilon_i) -> Memory3/1
  Memory3/1 -> [epsilon2]
  [T] -> Observer T#2/1(T)
  [epsilon] -> Observer T#2/2(epsilon)
  Differentiator2/1(Dx_d) -> Main Controller #2/2(DT_i)
  [x0] -> Module to compute Consensus Error #2/3(x0)
  [x_TP] -> Module to compute Consensus Error #2/2(x)
  Saturation/1 -> [u2_P], U2/1

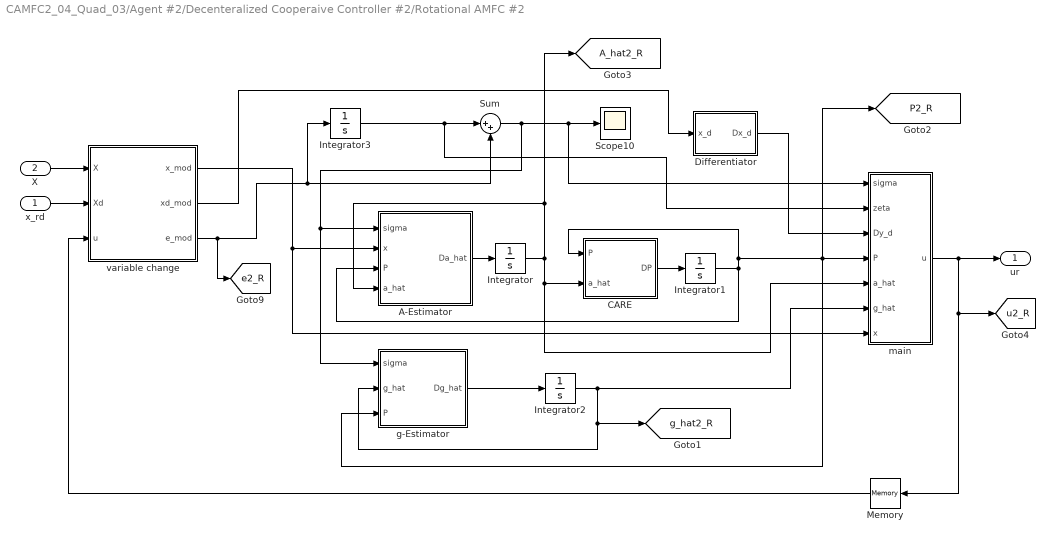
== system CAMFC2_04_Quad_03/Agent #2/Decenteralized Cooperaive Controller #2/Rotational AMFC #2 ==
  x_rd : Inport
  X : Inport  Port=2
  A-Estimator : MATLAB Function  TreatAsAtomicUnit=on
  CARE : MATLAB Function  TreatAsAtomicUnit=on
  Differentiator : Subsystem
  Integrator : Integrator  InitialCondition=zeros(n)
  Integrator1 : Integrator  InitialCondition=eye(n)
  Integrator2 : Integrator  InitialCondition=zeros(n,1)
  Integrator3 : Integrator  InitialCondition=zeros(n,1)
  Memory : Memory  InitialCondition=zeros(m,1)
  Scope10 : Scope
  Sum : Sum  Inputs=|++
  g-Estimator : MATLAB Function  TreatAsAtomicUnit=on
  main : MATLAB Function  TreatAsAtomicUnit=on
  variable change : MATLAB Function  TreatAsAtomicUnit=on
  ur : Outport
  tag scope: A_hat2_R=global, P2_R=global, e2_R=global, g_hat2_R=global, u2_R=global
  wires:
  Integrator2/1 -> g-Estimator/2(g_hat), [g_hat2_R], main/6(g_hat)
  Memory/1 -> variable change/3(u)
  variable change/3(e_mod) -> Integrator3/1, Sum/2, [e2_R]
  variable change/2(xd_mod) -> Differentiator/1(x_d)
  Integrator3/1 -> Sum/1, main/2(zeta)
  main/1(u) -> ur/1, [u2_R], Memory/1
  Differentiator/1(Dx_d) -> main/3(Dy_d)
  g-Estimator/1(Dg_hat) -> Integrator2/1
  Integrator/1 -> main/5(a_hat), CARE/2(a_hat), A-Estimator/4(a_hat), [A_hat2_R]
  Integrator1/1 -> main/4(P), g-Estimator/3(P), [P2_R], CARE/1(P), A-Estimator/3(P)
  variable change/1(x_mod) -> A-Estimator/2(x), main/7(x)
  A-Estimator/1(Da_hat) -> Integrator/1
  Sum/1 -> A-Estimator/1(sigma), g-Estimator/1(sigma), Scope10/1, main/1(sigma)
  CARE/1(DP) -> Integrator1/1
  X/1 -> variable change/1(X)
  x_rd/1 -> variable change/2(Xd)

== system CAMFC2_04_Quad_03/Agent #2/Decenteralized Cooperaive Controller #2/Velocity AMFC #2 ==
  x_rd : Inport
  X : Inport  Port=2
  "A-Estimator " : MATLAB Function  TreatAsAtomicUnit=on
  CARE : MATLAB Function  TreatAsAtomicUnit=on
  Differentiator : Subsystem
  Integrator : Integrator  InitialCondition=zeros(n0)
  Integrator1 : Integrator  InitialCondition=eye(n0)
  Integrator2 : Integrator  InitialCondition=zeros(n0,1)
  Integrator3 : Integrator  InitialCondition=zeros(n0,1)
  Sum : Sum  Inputs=|++
  g-Estimator : MATLAB Function  TreatAsAtomicUnit=on
  main : MATLAB Function  TreatAsAtomicUnit=on
  variable change : MATLAB Function  TreatAsAtomicUnit=on
  ut : Outport
  tag scope: A_hat2_V=global, P2_V=global, e2_V=global, g_hat2_V=global, u2_V=global
  wires:
  x_rd/1 -> variable change/2(Xd)
  X/1 -> variable change/1(X)
  CARE/1(DP) -> Integrator1/1
  Sum/1 -> main/1(sigma), g-Estimator/1(sigma), "A-Estimator "/1(sigma)
  "A-Estimator "/1(Da_hat) -> Integrator/1
  variable change/1(x_mod) -> main/7(x), "A-Estimator "/2(x)
  Integrator1/1 -> "A-Estimator "/3(P), CARE/1(P), [P2_V], g-Estimator/3(P), main/4(P)
  Integrator/1 -> [A_hat2_V], "A-Estimator "/4(a_hat), CARE/2(a_hat), main/5(a_hat)
  g-Estimator/1(Dg_hat) -> Integrator2/1
  Differentiator/1(Dx_d) -> main/3(Dy_d)
  main/1(u) -> ut/1, [u2_V]
  Integrator3/1 -> Sum/1, main/2(zeta)
  variable change/2(xd_mod) -> Differentiator/1(x_d)
  variable change/3(e_mod) -> Sum/2, Integrator3/1, [e2_V]
  Integrator2/1 -> main/6(g_hat), [g_hat2_V], g-Estimator/2(g_hat)

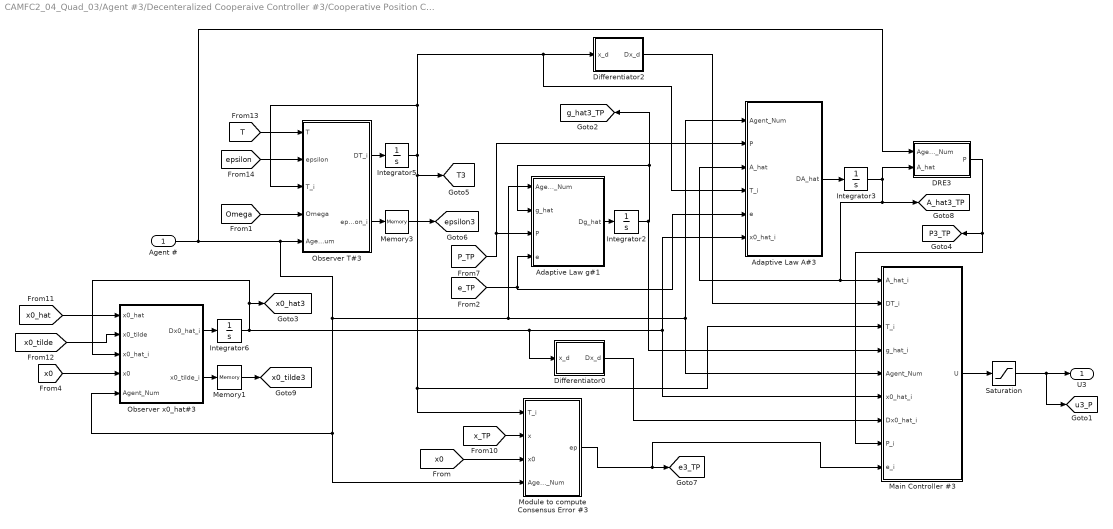
== system CAMFC2_04_Quad_03/Agent #3/Decenteralized Cooperaive Controller #3/Cooperative Position Controller #3 ==
  Agent # : Inport
  Adaptive Law A#3 : MATLAB Function  TreatAsAtomicUnit=on
  Adaptive Law g#1 : MATLAB Function  TreatAsAtomicUnit=on
  DRE3 : Subsystem
  Differentiator0 : Subsystem
  Differentiator2 : Subsystem
  Integrator2 : Integrator  InitialCondition=zeros(n0,1)
  Integrator3 : Integrator  InitialCondition=zeros(n0)
  Integrator5 : Integrator  InitialCondition=zeros(N+1,n0)
  Integrator6 : Integrator  InitialCondition=zeros(n0,1)
  Main Controller #3 : MATLAB Function  TreatAsAtomicUnit=on
  Memory1 : Memory  InitialCondition=zeros(n0,1)
  Memory3 : Memory  InitialCondition=zeros(N+1,n0)
  Module to compute Consensus Error #3 : MATLAB Function  TreatAsAtomicUnit=on
  Observer T#3 : MATLAB Function  TreatAsAtomicUnit=on
  Observer x0_hat#3 : MATLAB Function  TreatAsAtomicUnit=on
  Saturation : Saturate  UpperLimit=Vel_limit*ones(n0,1)  LowerLimit=-Vel_limit*ones(n0,1)
  U3 : Outport
  tag scope: A_hat3_TP=global, P3_TP=global, T3=global, e3_TP=global, epsilon3=global, g_hat3_TP=global, u3_P=global, x0_hat3=global, x0_tilde3=global
  wires:
  [x_TP] -> Module to compute Consensus Error #3/2(x)
  [x0] -> Module to compute Consensus Error #3/3(x0)
  Differentiator2/1(Dx_d) -> Main Controller #3/2(DT_i)
  [epsilon] -> Observer T#3/2(epsilon)
  [T] -> Observer T#3/1(T)
  Memory3/1 -> [epsilon3]
  Observer T#3/2(epsilon_i) -> Memory3/1
  Integrator5/1 -> [T3], Module to compute Consensus Error #3/1(T_i), Main Controller #3/3(T_i), Adaptive Law A#3/4(T_i), Differentiator2/1(x_d), Observer T#3/3(T_i)
  Observer T#3/1(DT_i) -> Integrator5/1
  Module to compute Consensus Error #3/1(ep) -> [e3_TP], Main Controller #3/9(e_i)
  Integrator3/1 -> DRE3/2(A_hat), [A_hat3_TP], Adaptive Law A#3/3(A_hat), Main Controller #3/1(A_hat_i)
  [e_TP] -> Adaptive Law A#3/5(e), Adaptive Law g#1/4(e)
  [P_TP] -> Adaptive Law A#3/2(P), Adaptive Law g#1/3(P)
  DRE3/1(P) -> Main Controller #3/8(P_i), [P3_TP]
  Integrator2/1 -> Main Controller #3/4(g_hat_i), Adaptive Law g#1/2(g_hat), [g_hat3_TP]
  Adaptive Law g#1/1(Dg_hat) -> Integrator2/1
  Adaptive Law A#3/1(DA_hat) -> Integrator3/1
  Agent #/1 -> DRE3/1(Agent_Num), Observer T#3/5(Agent_Num), Observer x0_hat#3/5(Agent_Num), Module to compute Consensus Error #3/4(Agent_Num), Adaptive Law g#1/1(Agent_Num), Adaptive Law A#3/1(Agent_Num), Main Controller #3/5(Agent_Num)
  Observer x0_hat#3/2(x0_tilde_i) -> Memory1/1
  Memory1/1 -> [x0_tilde3]
  Observer x0_hat#3/1(Dx0_hat_i) -> Integrator6/1
  [x0_tilde] -> Observer x0_hat#3/2(x0_tilde)
  [x0] -> Observer x0_hat#3/4(x0)
  [x0_hat] -> Observer x0_hat#3/1(x0_hat)
  Integrator6/1 -> Observer x0_hat#3/3(x0_hat_i), [x0_hat3], Differentiator0/1(x_d), Main Controller #3/6(x0_hat_i), Adaptive Law A#3/6(x0_hat_i)
  Differentiator0/1(Dx_d) -> Main Controller #3/7(Dx0_hat_i)
  [Omega] -> Observer T#3/4(Omega)
  Main Controller #3/1(U) -> Saturation/1
  Saturation/1 -> U3/1, [u3_P]

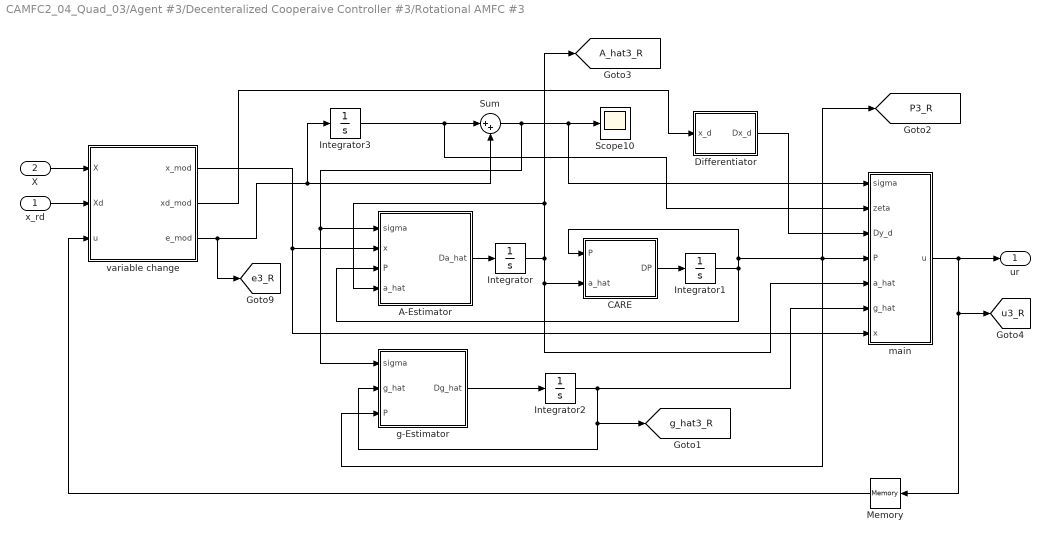
== system CAMFC2_04_Quad_03/Agent #3/Decenteralized Cooperaive Controller #3/Rotational AMFC #3 ==
  x_rd : Inport
  X : Inport  Port=2
  A-Estimator : MATLAB Function  TreatAsAtomicUnit=on
  CARE : MATLAB Function  TreatAsAtomicUnit=on
  Differentiator : Subsystem
  Integrator : Integrator  InitialCondition=zeros(n)
  Integrator1 : Integrator  InitialCondition=eye(n)
  Integrator2 : Integrator  InitialCondition=zeros(n,1)
  Integrator3 : Integrator  InitialCondition=zeros(n,1)
  Memory : Memory  InitialCondition=zeros(m,1)
  Scope10 : Scope
  Sum : Sum  Inputs=|++
  g-Estimator : MATLAB Function  TreatAsAtomicUnit=on
  main : MATLAB Function  TreatAsAtomicUnit=on
  variable change : MATLAB Function  TreatAsAtomicUnit=on
  ur : Outport
  tag scope: A_hat3_R=global, P3_R=global, e3_R=global, g_hat3_R=global, u3_R=global
  wires:
  x_rd/1 -> variable change/2(Xd)
  X/1 -> variable change/1(X)
  CARE/1(DP) -> Integrator1/1
  Sum/1 -> main/1(sigma), Scope10/1, g-Estimator/1(sigma), A-Estimator/1(sigma)
  A-Estimator/1(Da_hat) -> Integrator/1
  variable change/1(x_mod) -> main/7(x), A-Estimator/2(x)
  Integrator1/1 -> A-Estimator/3(P), CARE/1(P), [P3_R], g-Estimator/3(P), main/4(P)
  Integrator/1 -> [A_hat3_R], A-Estimator/4(a_hat), CARE/2(a_hat), main/5(a_hat)
  g-Estimator/1(Dg_hat) -> Integrator2/1
  Differentiator/1(Dx_d) -> main/3(Dy_d)
  main/1(u) -> Memory/1, [u3_R], ur/1
  Integrator3/1 -> main/2(zeta), Sum/1
  variable change/2(xd_mod) -> Differentiator/1(x_d)
  variable change/3(e_mod) -> [e3_R], Sum/2, Integrator3/1
  Memory/1 -> variable change/3(u)
  Integrator2/1 -> main/6(g_hat), [g_hat3_R], g-Estimator/2(g_hat)

== system CAMFC2_04_Quad_03/Agent #3/Decenteralized Cooperaive Controller #3/Velocity AMFC #3 ==
  x_rd : Inport
  X : Inport  Port=2
  "A-Estimator " : MATLAB Function  TreatAsAtomicUnit=on
  CARE : MATLAB Function  TreatAsAtomicUnit=on
  Differentiator : Subsystem
  Integrator : Integrator  InitialCondition=zeros(n0)
  Integrator1 : Integrator  InitialCondition=eye(n0)
  Integrator2 : Integrator  InitialCondition=zeros(n0,1)
  Integrator3 : Integrator  InitialCondition=zeros(n0,1)
  Sum : Sum  Inputs=|++
  g-Estimator : MATLAB Function  TreatAsAtomicUnit=on
  main : MATLAB Function  TreatAsAtomicUnit=on
  variable change : MATLAB Function  TreatAsAtomicUnit=on
  ur : Outport
  tag scope: A_hat3_V=global, P3_V=global, e3_V=global, g_hat3_V=global, u3_V=global
  wires:
  Integrator2/1 -> g-Estimator/2(g_hat), [g_hat3_V], main/6(g_hat)
  variable change/3(e_mod) -> [e3_V], Integrator3/1, Sum/2
  variable change/2(xd_mod) -> Differentiator/1(x_d)
  Integrator3/1 -> Sum/1, main/2(zeta)
  main/1(u) -> [u3_V], ur/1
  Differentiator/1(Dx_d) -> main/3(Dy_d)
  g-Estimator/1(Dg_hat) -> Integrator2/1
  Integrator/1 -> main/5(a_hat), CARE/2(a_hat), "A-Estimator "/4(a_hat), [A_hat3_V]
  Integrator1/1 -> main/4(P), g-Estimator/3(P), [P3_V], CARE/1(P), "A-Estimator "/3(P)
  variable change/1(x_mod) -> "A-Estimator "/2(x), main/7(x)
  "A-Estimator "/1(Da_hat) -> Integrator/1
  Sum/1 -> "A-Estimator "/1(sigma), g-Estimator/1(sigma), main/1(sigma)
  CARE/1(DP) -> Integrator1/1
  X/1 -> variable change/1(X)
  x_rd/1 -> variable change/2(Xd)

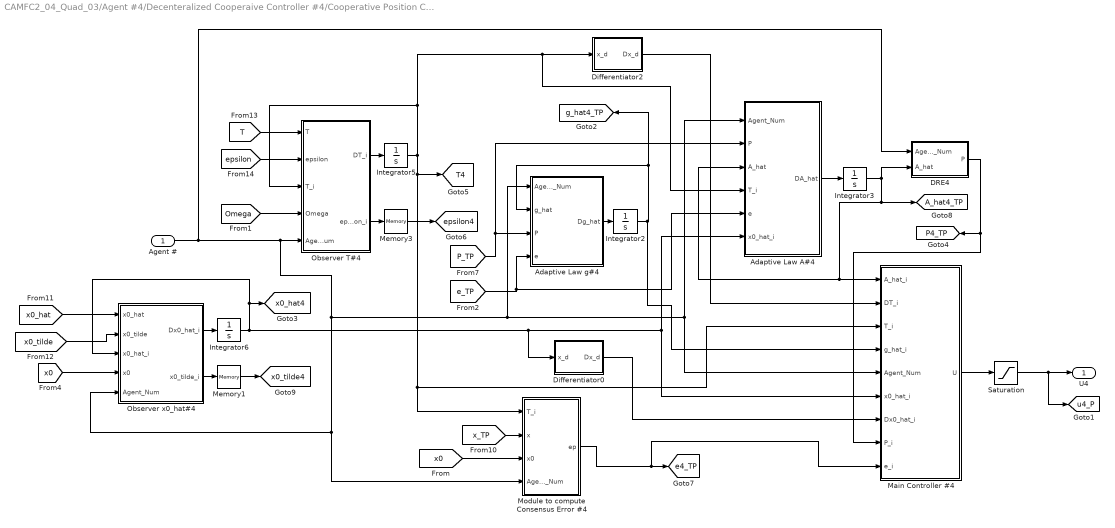
== system CAMFC2_04_Quad_03/Agent #4/Decenteralized Cooperaive Controller #4/Cooperative Position Controller #4 ==
  Agent # : Inport
  Adaptive Law A#4 : MATLAB Function  TreatAsAtomicUnit=on
  Adaptive Law g#4 : MATLAB Function  TreatAsAtomicUnit=on
  DRE4 : Subsystem
  Differentiator0 : Subsystem
  Differentiator2 : Subsystem
  Integrator2 : Integrator  InitialCondition=zeros(n0,1)
  Integrator3 : Integrator  InitialCondition=zeros(n0)
  Integrator5 : Integrator  InitialCondition=zeros(N+1,n0)
  Integrator6 : Integrator  InitialCondition=zeros(n0,1)
  Main Controller #4 : MATLAB Function  TreatAsAtomicUnit=on
  Memory1 : Memory  InitialCondition=zeros(n0,1)
  Memory3 : Memory  InitialCondition=zeros(N+1,n0)
  Module to compute Consensus Error #4 : MATLAB Function  TreatAsAtomicUnit=on
  Observer T#4 : MATLAB Function  TreatAsAtomicUnit=on
  Observer x0_hat#4 : MATLAB Function  TreatAsAtomicUnit=on
  Saturation : Saturate  UpperLimit=Vel_limit*ones(n0,1)  LowerLimit=-Vel_limit*ones(n0,1)
  U4 : Outport
  tag scope: A_hat4_TP=global, P4_TP=global, T4=global, e4_TP=global, epsilon4=global, g_hat4_TP=global, u4_P=global, x0_hat4=global, x0_tilde4=global
  wires:
  Main Controller #4/1(U) -> Saturation/1
  [Omega] -> Observer T#4/4(Omega)
  Differentiator0/1(Dx_d) -> Main Controller #4/7(Dx0_hat_i)
  Integrator6/1 -> Differentiator0/1(x_d), Adaptive Law A#4/6(x0_hat_i), Main Controller #4/6(x0_hat_i), [x0_hat4], Observer x0_hat#4/3(x0_hat_i)
  [x0_hat] -> Observer x0_hat#4/1(x0_hat)
  [x0] -> Observer x0_hat#4/4(x0)
  [x0_tilde] -> Observer x0_hat#4/2(x0_tilde)
  Observer x0_hat#4/1(Dx0_hat_i) -> Integrator6/1
  Memory1/1 -> [x0_tilde4]
  Observer x0_hat#4/2(x0_tilde_i) -> Memory1/1
  Agent #/1 -> Main Controller #4/5(Agent_Num), Adaptive Law A#4/1(Agent_Num), Adaptive Law g#4/1(Agent_Num), Module to compute Consensus Error #4/4(Agent_Num), Observer x0_hat#4/5(Agent_Num), Observer T#4/5(Agent_Num), DRE4/1(Agent_Num)
  Adaptive Law A#4/1(DA_hat) -> Integrator3/1
  Adaptive Law g#4/1(Dg_hat) -> Integrator2/1
  Integrator2/1 -> [g_hat4_TP], Adaptive Law g#4/2(g_hat), Main Controller #4/4(g_hat_i)
  DRE4/1(P) -> [P4_TP], Main Controller #4/8(P_i)
  [P_TP] -> Adaptive Law g#4/3(P), Adaptive Law A#4/2(P)
  [e_TP] -> Adaptive Law g#4/4(e), Adaptive Law A#4/5(e)
  Integrator3/1 -> Main Controller #4/1(A_hat_i), Adaptive Law A#4/3(A_hat), [A_hat4_TP], DRE4/2(A_hat)
  Module to compute Consensus Error #4/1(ep) -> Main Controller #4/9(e_i), [e4_TP]
  Observer T#4/1(DT_i) -> Integrator5/1
  Integrator5/1 -> Observer T#4/3(T_i), Differentiator2/1(x_d), Adaptive Law A#4/4(T_i), Main Controller #4/3(T_i), Module to compute Consensus Error #4/1(T_i), [T4]
  Observer T#4/2(epsilon_i) -> Memory3/1
  Memory3/1 -> [epsilon4]
  [T] -> Observer T#4/1(T)
  [epsilon] -> Observer T#4/2(epsilon)
  Differentiator2/1(Dx_d) -> Main Controller #4/2(DT_i)
  [x0] -> Module to compute Consensus Error #4/3(x0)
  [x_TP] -> Module to compute Consensus Error #4/2(x)
  Saturation/1 -> [u4_P], U4/1

== system CAMFC2_04_Quad_03/Agent #4/Decenteralized Cooperaive Controller #4/Rotational AMFC #4 ==
  x_rd : Inport
  X : Inport  Port=2
  A-Estimator : MATLAB Function  TreatAsAtomicUnit=on
  CARE : MATLAB Function  TreatAsAtomicUnit=on
  Differentiator : Subsystem
  Integrator : Integrator  InitialCondition=zeros(n)
  Integrator1 : Integrator  InitialCondition=eye(n)
  Integrator2 : Integrator  InitialCondition=zeros(n,1)
  Integrator3 : Integrator  InitialCondition=zeros(n,1)
  Memory : Memory  InitialCondition=zeros(m,1)
  Scope10 : Scope
  Sum : Sum  Inputs=|++
  g-Estimator : MATLAB Function  TreatAsAtomicUnit=on
  main : MATLAB Function  TreatAsAtomicUnit=on
  variable change : MATLAB Function  TreatAsAtomicUnit=on
  ur : Outport
  tag scope: A_hat4_R=global, P4_R=global, e4_R=global, g_hat4_R=global, u4_R=global
  wires:
  Integrator2/1 -> g-Estimator/2(g_hat), [g_hat4_R], main/6(g_hat)
  Memory/1 -> variable change/3(u)
  variable change/3(e_mod) -> Integrator3/1, Sum/2, [e4_R]
  variable change/2(xd_mod) -> Differentiator/1(x_d)
  Integrator3/1 -> Sum/1, main/2(zeta)
  main/1(u) -> ur/1, [u4_R], Memory/1
  Differentiator/1(Dx_d) -> main/3(Dy_d)
  g-Estimator/1(Dg_hat) -> Integrator2/1
  Integrator/1 -> main/5(a_hat), CARE/2(a_hat), A-Estimator/4(a_hat), [A_hat4_R]
  Integrator1/1 -> main/4(P), g-Estimator/3(P), [P4_R], CARE/1(P), A-Estimator/3(P)
  variable change/1(x_mod) -> A-Estimator/2(x), main/7(x)
  A-Estimator/1(Da_hat) -> Integrator/1
  Sum/1 -> A-Estimator/1(sigma), g-Estimator/1(sigma), Scope10/1, main/1(sigma)
  CARE/1(DP) -> Integrator1/1
  X/1 -> variable change/1(X)
  x_rd/1 -> variable change/2(Xd)

== system CAMFC2_04_Quad_03/Agent #4/Decenteralized Cooperaive Controller #4/Velocity AMFC #4 ==
  x_rd : Inport
  X : Inport  Port=2
  "A-Estimator " : MATLAB Function  TreatAsAtomicUnit=on
  CARE : MATLAB Function  TreatAsAtomicUnit=on
  Differentiator : Subsystem
  Integrator : Integrator  InitialCondition=zeros(n0)
  Integrator1 : Integrator  InitialCondition=eye(n0)
  Integrator2 : Integrator  InitialCondition=zeros(n0,1)
  Integrator3 : Integrator  InitialCondition=zeros(n0,1)
  Sum : Sum  Inputs=|++
  g-Estimator : MATLAB Function  TreatAsAtomicUnit=on
  main : MATLAB Function  TreatAsAtomicUnit=on
  variable change : MATLAB Function  TreatAsAtomicUnit=on
  ur : Outport
  tag scope: A_hat4_V=global, P4_V=global, e4_V=global, g_hat4_V=global, u4_V=global
  wires:
  x_rd/1 -> variable change/2(Xd)
  X/1 -> variable change/1(X)
  CARE/1(DP) -> Integrator1/1
  Sum/1 -> main/1(sigma), g-Estimator/1(sigma), "A-Estimator "/1(sigma)
  "A-Estimator "/1(Da_hat) -> Integrator/1
  variable change/1(x_mod) -> main/7(x), "A-Estimator "/2(x)
  Integrator1/1 -> "A-Estimator "/3(P), CARE/1(P), [P4_V], g-Estimator/3(P), main/4(P)
  Integrator/1 -> [A_hat4_V], "A-Estimator "/4(a_hat), CARE/2(a_hat), main/5(a_hat)
  g-Estimator/1(Dg_hat) -> Integrator2/1
  Differentiator/1(Dx_d) -> main/3(Dy_d)
  main/1(u) -> ur/1, [u4_V]
  Integrator3/1 -> main/2(zeta), Sum/1
  variable change/2(xd_mod) -> Differentiator/1(x_d)
  variable change/3(e_mod) -> Sum/2, Integrator3/1, [e4_V]
  Integrator2/1 -> main/6(g_hat), [g_hat4_V], g-Estimator/2(g_hat)

== system CAMFC2_04_Quad_03/Data Bus /Observers Log/For matrix Plot10 ==
  T : Inport
  MATLAB Function : MATLAB Function  TreatAsAtomicUnit=on
  To Workspace : ToWorkspace  VariableName=T3  SaveFormat=Structure With Time  SampleTime=-1
  wires:
  T/1 -> MATLAB Function/1(u)
  MATLAB Function/1(y) -> To Workspace/1
